simulink model "ALGO_Corner_TrajTrack_MPC_T1_SP_LTR"  (Simulink 9.3)
settings: Solver=VariableStepAuto  StartTime=0.0  StopTime=12  RelTol=1e-3
libraries: simulink x7, Solver_SF x1
settings Model: Creator=QXJ  LastModifiedBy=QXJ
settings DataIOCC: SaveFormat=Dataset  SignalLoggingSaveFormat=Dataset  ReturnWorkspaceOutputs=on
settings OptimizationCC: LifeSpan=auto
settings DebuggingCC: UnderspecifiedInitializationDetection=Simplified  MergeDetectMultiDrivingBlocksExec=error  FcnCallInpInsideContextMsg=error  SFUnexpectedBacktrackingDiag=error  SFNoUnconditionalDefaultTransitionDiag=error  SFExecutionAtInitializationDiag=warning  ArithmeticOperatorsInVariantConditions=error
settings HardwareCC: ProdBitPerPointer=64  ProdBitPerSizeT=64  ProdBitPerPtrDiffT=64  ProdLargestAtomicFloat=Float  ProdIntDivRoundTo=Zero  ProdEndianess=LittleEndian  ProdWordSize=64  ProdHWDeviceType=Intel->x86-64 (Windows64)
settings ModelReferenceCC: PropagateSignalLabelsOutOfModel=on
settings SFSimCC: SimUseLocalCustomCode=on
settings RTWCC: RTWUseLocalCustomCode=on
settings CodeAppCC: StateflowObjectComments=off
settings GRTTargetCC: TargetLangStandard=C99 (ISO)  CombineOutputUpdateFcns=on  GRTInterface=off
settings ConfigComp: CovMetricSettings=dwe  CovHtmlReporting=off  CovSaveCumulativeToWorkspaceVar=off  CovSaveSingleToWorkspaceVar=off  CovExternalEMLEnable=on

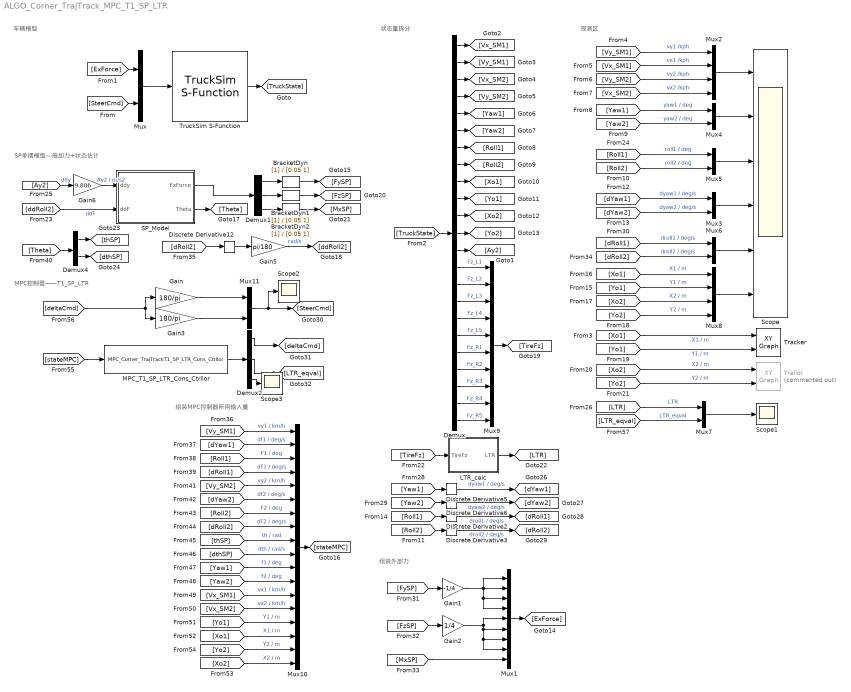
== system ALGO_Corner_TrajTrack_MPC_T1_SP_LTR ==
  note: MPC控制器——T1_SP_LTR
  note: 组装MPC控制器所用输入量
  note: 观测区
  note: 车辆模型
  note: 组装外部力
  note: SP单摆模型---施加力+状态估计
  note: 状态量拆分
  BracketDyn : TransferFcn  Denominator=[0.05 1]
  BracketDyn1 : TransferFcn  Denominator=[0.05 1]
  BracketDyn2 : TransferFcn  Denominator=[0.05 1]
  Demux : Demux  Outputs=23
  Demux1 : Demux  Outputs=3
  Demux2 : Demux  Outputs=3
  Demux4 : Demux  Outputs=2
  Discrete Derivative{2..3,5..6,12} (5 alike) : simulink/Discrete/Discrete Derivative  gainval=1.0  ICPrevScaledInput=0.0  OutMin=[]  OutMax=[]  OutDataType=fixdt(1, 16)  OutScaling=2^-10  DoSatur=off
  Gain : Gain  Gain=180/pi
  Gain1 : Gain  Gain=-1/4
  Gain2 : Gain  Gain=1/4
  Gain3 : Gain  Gain=180/pi
  Gain5 : Gain  Gain=pi/180
  Gain6 : Gain  Gain=9.806
  "LTR_calc " : MATLAB Function  TreatAsAtomicUnit=on
  MPC_T1_SP_LTR_Cons_Ctrllor : S-Function  FunctionName=MPC_Corner_TrajTrackT1_SP_LTR_Cons_Ctrllor  SFunctionDeploymentMode=off  EnableBusSupport=off
  Mux{,3..7,11} (7 alike) : Mux  Inputs=2
  Mux1 : Mux  Inputs=9
  Mux10 : Mux  Inputs=18
  Mux2 : Mux
  Mux8 : Mux
  Mux9 : Mux  Inputs=10
  SP_Model : MATLAB Function  TreatAsAtomicUnit=on  SystemSampleTime=0.005
  Scope : Scope  NumInputPorts=6
  Scope1 : Scope
  Scope2 : Scope
  Scope3 : Scope
  Tracker : simulink/Sinks/XY Graph  xmin=-10  xmax=80  ymin=-10  ymax=80  st=-1
  "Trailor " : simulink/Sinks/XY Graph  Commented=on  xmin=-10  xmax=250  ymin=-20  ymax=20  st=-1
  TruckSim S-Function : Solver_SF/TruckSim S-Function  Priority=1  SIMFILE=ALGO_Corner_Tanker_TrajTrack_MPC_T1_SP_LTR.sim
  wires:
  TruckSim S-Function/1 -> [TruckState]
  Mux/1 -> TruckSim S-Function/1
  [MxSP] -> Mux1/9
  Discrete Derivative12/1 -> Gain5/1
  Demux4/2 -> [dthSP]
  Demux4/1 -> [thSP]
  [Theta] -> Demux4/1
  [FySP] -> Gain1/1
  Gain6/1 -> SP_Model/1(ddy)  "Ay2 / m/s2"
  Gain5/1 -> [ddRoll2]  "rad/s"
  Gain2/1 -> Mux1/5, Mux1/6, Mux1/7, Mux1/8
  [FzSP] -> Gain2/1
  Gain1/1 -> Mux1/2, Mux1/3, Mux1/4, Mux1/1
  [dRoll2] -> Discrete Derivative12/1
  [ddRoll2] -> SP_Model/2(ddF)  "ddF"
  BracketDyn/1 -> [FySP]
  BracketDyn1/1 -> [FzSP]
  BracketDyn2/1 -> [MxSP]
  SP_Model/1(ExForce) -> Demux1/1
  [Ay2] -> Gain6/1  "ddy"
  Demux1/1 -> BracketDyn/1
  Demux1/2 -> BracketDyn1/1
  Demux1/3 -> BracketDyn2/1
  SP_Model/2(Theta) -> [Theta]
  Mux1/1 -> [ExForce]
  [Yo1] -> Mux8/2  "Y1 / m"
  [Roll1] -> Mux5/1  "roll1 / deg"
  Mux3/1 -> Scope/4
  [Vx_SM1] -> Mux2/2  "vx1 /kph"
  [dRoll1] -> Mux6/1  "droll1 / deg/s"
  [Xo1] -> Tracker/1  "X1 / m"
  [Roll2] -> Mux5/2  "roll2 / deg"
  Mux8/1 -> Scope/6
  [Yo1] -> Tracker/2  "Y1 / m"
  Mux6/1 -> Scope/5
  Mux2/1 -> Scope/1
  [Yo2] -> "Trailor "/2  "Y2 / m"
  [dYaw2] -> Mux3/2  "dyaw2 / deg/s"
  [Yaw2] -> Mux4/2  "yaw2 / deg"
  [Vx_SM2] -> Mux2/4  "vx2 /kph"
  Mux5/1 -> Scope/3
  [Xo1] -> Mux8/1  "X1 / m"
  [Yaw1] -> Mux4/1  "yaw1 / deg"
  [Vy_SM2] -> Mux2/3  "vy2 /kph"
  [dYaw1] -> Mux3/1  "dyaw1 / deg/s"
  [Yo2] -> Mux8/4  "Y2 / m"
  Mux4/1 -> Scope/2
  [Xo2] -> Mux8/3  "X2 / m"
  [Xo2] -> "Trailor "/1  "X2 / m"
  [Vy_SM1] -> Mux2/1  "vy1 /kph"
  [dRoll2] -> Mux6/2  "droll2 / deg/s"
  Demux/13 -> [Ay2]
  Demux/8 -> [Roll2]
  Demux/6 -> [Yaw2]
  Demux/2 -> [Vy_SM1]
  Demux/4 -> [Vy_SM2]
  Demux/9 -> [Xo1]
  Demux/10 -> [Yo1]
  Demux/11 -> [Xo2]
  Demux/7 -> [Roll1]
  Demux/5 -> [Yaw1]
  Demux/1 -> [Vx_SM1]
  Demux/3 -> [Vx_SM2]
  Demux/12 -> [Yo2]
  [TruckState] -> Demux/1
  Demux/14 -> Mux9/1  "Fz_L1"
  Demux/15 -> Mux9/2  "Fz_L2"
  Demux/16 -> Mux9/3  "Fz_L3"
  Demux/17 -> Mux9/4  "Fz_L4"
  Demux/18 -> Mux9/5  "Fz_L5"
  Demux/19 -> Mux9/6  "Fz_R1"
  Demux/20 -> Mux9/7  "Fz_R2"
  Demux/21 -> Mux9/8  "Fz_R3"
  Demux/22 -> Mux9/9  "Fz_R4"
  Demux/23 -> Mux9/10  "Fz_R5"
  Mux9/1 -> [TireFz]
  [TireFz] -> "LTR_calc "/1(TireFz)
  "LTR_calc "/1(LTR) -> [LTR]
  [Yaw2] -> Discrete Derivative6/1
  Discrete Derivative5/1 -> [dYaw1]  "dyaw1 / deg/s"
  [Yaw1] -> Discrete Derivative5/1
  Discrete Derivative6/1 -> [dYaw2]  "dyaw2 / deg/s"
  [Roll1] -> Discrete Derivative2/1
  [Roll2] -> Discrete Derivative3/1
  Discrete Derivative2/1 -> [dRoll1]  "droll1 / deg/s"
  Discrete Derivative3/1 -> [dRoll2]  "droll2 / deg/s"
  [ExForce] -> Mux/1
  [SteerCmd] -> Mux/2
  [Vy_SM1] -> Mux10/1  "vy1 / km/h"
  [dYaw1] -> Mux10/2  "df1 / deg/s"
  [Roll1] -> Mux10/3  "F1 / deg"
  [dRoll1] -> Mux10/4  "dF1 / deg/s"
  [Vy_SM2] -> Mux10/5  "vy2 / km/h"
  [dYaw2] -> Mux10/6  "df2 / deg/s"
  [Roll2] -> Mux10/7  "F2 / deg"
  [dRoll2] -> Mux10/8  "dF2 / deg/s"
  [thSP] -> Mux10/9  "th / rad"
  [dthSP] -> Mux10/10  "dth / rad/s"
  [Yaw1] -> Mux10/11  "f1 / deg"
  [Yaw2] -> Mux10/12  "f2 / deg"
  [Vx_SM1] -> Mux10/13  "vx1 / km/h"
  [Vx_SM2] -> Mux10/14  "vx2 / km/h"
  [Xo2] -> Mux10/18  "X2 / m"
  [Yo2] -> Mux10/17  "Y2 / m"
  [Xo1] -> Mux10/16  "X1 / m"
  [Yo1] -> Mux10/15  "Y1 / m"
  Mux10/1 -> [stateMPC]
  [stateMPC] -> MPC_T1_SP_LTR_Cons_Ctrllor/1
  MPC_T1_SP_LTR_Cons_Ctrllor/1 -> Demux2/1
  Mux11/1 -> Scope2/1, [SteerCmd]
  Demux2/1 -> [deltaCmd]
  Gain/1 -> Mux11/1
  Gain3/1 -> Mux11/2
  [deltaCmd] -> Gain3/1, Gain/1
  Demux2/2 -> [LTR_eqval]
  [LTR] -> Mux7/1  "LTR"
  [LTR_eqval] -> Mux7/2  "LTR_eqval"
  Mux7/1 -> Scope1/1
  Demux2/3 -> Scope3/1

== matlab function SP_Model ==
  data: ddy input double; ExForce output double; ddF input double; Theta output double
function [ExForce,Theta] = SP_Model(ddy,ddF)
persistent sim_param Ts y0
%% 定义摆
if isempty(Ts)
%SP模型，共5个参数拟合
% 参数 m1 h0 hp lp coeff
x=[10890,1.5,0.13,0.97,0.13];
% 获取参数
sim_param=getParam_SP(x);
%初始状态量
y0=zeros(9,1);
%采样时间
Ts=0.005;
end

y=y0;

%% 求解微分方程
dy=zeros(9,1);
dy(1)=y(2);
dy(2)=ddy;
dy(3)=(dy(2)-y(3))/Ts;
dy(4)=y(5);
dy(5)=ddF;
dy(6)=(dy(5)-y(6))/Ts;
dy(7)=y(8);
dy(8)=calc_ddth_SP(y,sim_param);
dy(9)=(dy(8)-y(9))/Ts;
y=y0+dy*Ts;
%% 计算三向力输出
[Fy,Fz,Mx]=calc_Fp_SP(y,sim_param);
ExForce=[Fy,Fz,Mx];
%% 更新状态量
y0=y;
th=y(7);
dth=y(8);
Theta=[th,dth];
end

%% 根据变量获取参数
function sim_param=getParam_SP(x)
%根据变量生成传输参数
TotMass=14462;
m1=x(1);%参数1
m0=TotMass-m1;
h0=x(2);%参数2
hp=x(3);%参数3
lp=x(4);%参数4
g=9.806;
coeff=x(5);%参数5
sim_param=[m0,m1,h0,hp,lp,g,coeff];
end

%% 求解三向力输出
function [Fy,Fz,Mx] = calc_Fp_SP(state,param)
% sim_param=[m0,m1,h0,hp,lp,g,coeff];
m0=param(1);
m1=param(2);
h0=param(3);
hp=param(4);
lp=param(5);
g=param(6);
% co=param(7);

% y=state(1);
% dy=state(2);
ddy=state(3);
f=state(4);
df=state(5);
ddf=state(6);
th=state(7);
dth=state(8);
ddth=state(9);

%定义运算符简写
sf=sin(f);
cf=cos(f);
s2=sin(th+f);
c2=cos(th+f);
L=lp+hp;
%定义质量块的 位置矢量
exh=0.77; %额外增加的高度是罐底到车轴心的高度
R0=[-(exh+h0)*sf,(exh+h0)*cf];

R1=[-(exh+L)*sf+lp*s2
    (exh+L)*cf-lp*c2];

ddRp0=[ddy-h0*cf*ddf+df^2*h0*sf
-h0*sf*ddf-h0*cf*df^2+g];

ddRp1=[ddy+ddf*(-L*cf+lp*c2)+ddth*(lp*c2)+df^2*(L*sf-lp*s2)+dth^2*(-lp*s2)+df*dth*(-2*lp*s2)
ddf*(-L*sf+lp*s2)+ddth*(lp*s2)+df^2*(-L*cf+lp*c2)+dth^2*(lp*c2)+df*dth*(2*lp*c2)+g];

Fp=m0*ddRp0+m1*ddRp1;
Fy=Fp(1)*cf-(-Fp(2))*sf;
Fz=(-Fp(2))*cf+Fp(1)*sf;
Mx0=(m0*(R0(1)*-ddRp0(2)+R0(2)*ddRp0(1)));
Mx1=(m1*(R1(1)*-ddRp1(2)+R1(2)*ddRp1(1)));

Mx=Mx0+Mx1;

end
%% 求解ddth
function ddth = calc_ddth_SP(state,param)
% sim_param=[m0,m1,h0,hp,lp,g,coeff];
% m0=param(1);
% m1=param(2);
% h0=param(3);
hp=param(4);
lp=param(5);
g=param(6);
co=param(7);

% y=state(1);
% dy=state(2);
ddy=state(3);
f=state(4);
df=state(5);
ddf=state(6);
th=state(7);
dth=state(8);
% ddth=state(9);


%定义运算符简写
s1=sin(th);
c1=cos(th);
s2=sin(th+f);
c2=cos(th+f);
L=lp+hp;

ddth=-(ddy*lp*c2+ddf*(-lp*L*c1+lp^2)-df^2*lp*L*s1+g*lp*s2)/(lp^2);
ddth=ddth-co*dth;

end

== matlab function LTR_calc  ==
  data: TireFz input double; LTR output double
function LTR = fcn(TireFz)
% 分配物理量
FzL=sum(TireFz(1:5));
FzR=sum(TireFz(6:10));
% 进行计算
LTR=(FzL-FzR)/(FzL+FzR);
end
